simulink library "simpSubPlatform_cl"  (R2018b)
settings: Solver=VariableStepAuto  StartTime=0.0  StopTime=10.0  RelTol=1e-3
values from neighbouring files (symbols this model uses):
  CB2CMVec = [0 0 0]    [simpSubPlatform_ts.m]
  grav = 9.81    [simpSubPlatform_ts.m]
  inertiaMatrix = eye(3)    [simpSubPlatform_ts.m]
  initAngVel = [0 0 0]    [simpSubPlatform_ts.m]
  initEulerAngles = [0 0 0]    [simpSubPlatform_ts.m]
  initPos = [0 0 100]    [simpSubPlatform_ts.m]
  initVel = [0 0 0]    [simpSubPlatform_ts.m]
  m = mass    (= 2692.30769231)    [simpSubPlatform_ts.m]
  rho = 1000    [simpSubPlatform_ts.m]
  thr1Pt = [0 1 -.5]    [simpSubPlatform_ts.m]
  thr2Pt = [cosd(30),-sind(30),-.5]    [simpSubPlatform_ts.m]
  thr3Pt = [-cosd(30),-sind(30),-.5]    [simpSubPlatform_ts.m]
  vol = 3.5    [simpSubPlatform_ts.m]
undefined symbols (not defined in the file or in its folder): initAngRates, Jinv, sixDoFDynamics, sixDoFDynamics_ul
libraries: vrlib x5, eulAng2RotMat_ul x1
settings Model: Creator=Erin B  LastModifiedBy=Erin B

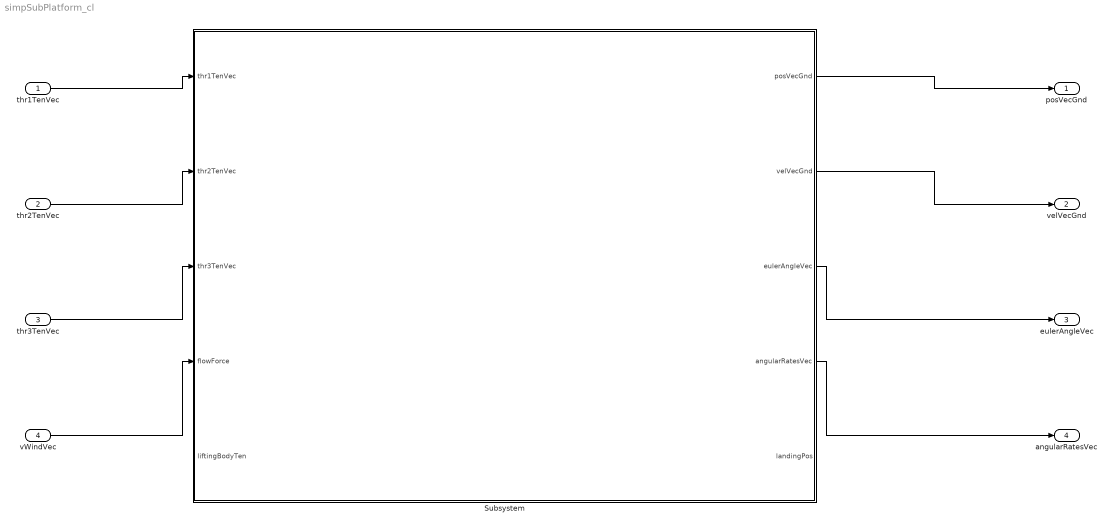
== system simpSubPlatform_cl ==
  thr1TenVec : Inport
  thr2TenVec : Inport  Port=2
  thr3TenVec : Inport  Port=3
  vWindVec : Inport  Port=4
  Subsystem : Subsystem
  posVecGnd : Outport
  velVecGnd : Outport  Port=2
  eulerAngleVec : Outport  Port=3
  angularRatesVec : Outport  Port=4
  wires:
  thr1TenVec/1 -> Subsystem/1(thr1TenVec)
  thr2TenVec/1 -> Subsystem/2(thr2TenVec)
  thr3TenVec/1 -> Subsystem/3(thr3TenVec)
  vWindVec/1 -> Subsystem/4(flowForce)
  Subsystem/1(posVecGnd) -> posVecGnd/1
  Subsystem/2(velVecGnd) -> velVecGnd/1
  Subsystem/3(eulerAngleVec) -> eulerAngleVec/1
  Subsystem/4(angularRatesVec) -> angularRatesVec/1

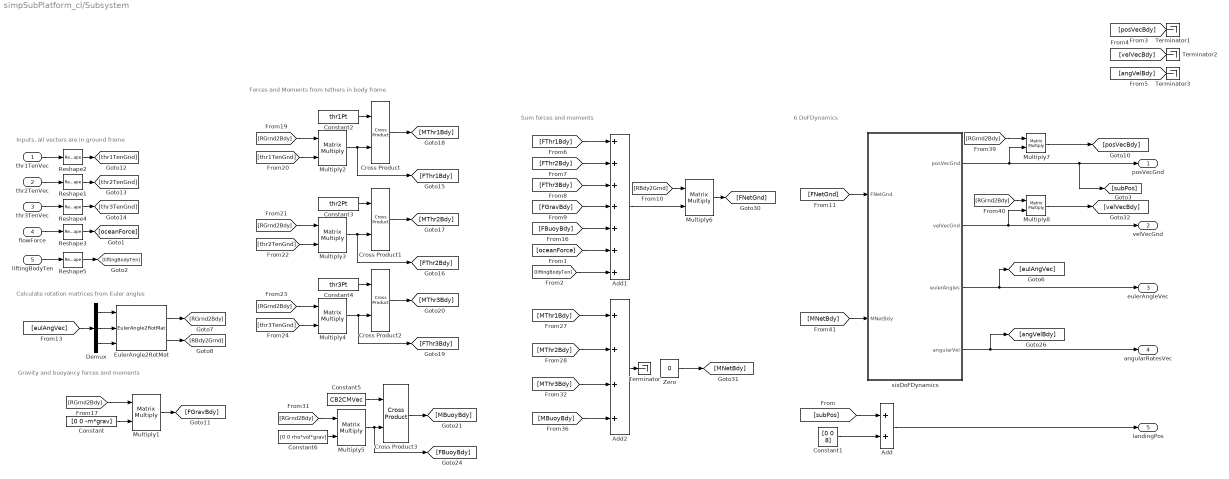
== system simpSubPlatform_cl/Subsystem ==
  note: Inputs, all vectors are in ground frame
  note: Calculate rotation matrices from Euler angles
  note: Gravity and buoyancy forces and moments
  note: Forces and Moments from tethers in body frame
  note: Sum forces and moments
  note: 6 DoFDynamics
  thr1TenVec : Inport
  thr2TenVec : Inport  Port=2
  thr3TenVec : Inport  Port=3
  flowForce : Inport  Port=4
  liftingBodyTen : Inport  Port=5
  Add : Sum
  Add1 : Sum  Inputs=+++++++
  Add2 : Sum  Inputs=++++
  Constant : Constant  Value=[0 0 -m*grav]
  Constant1 : Constant  Value=[0 0 8]
  Constant2 : Constant  Value=thr1Pt
  Constant3 : Constant  Value=thr2Pt
  Constant4 : Constant  Value=thr3Pt
  Constant5 : Constant  Value=CB2CMVec
  Constant6 : Constant  Value=[0 0 rho*vol*grav]
  Cross Product{,1..3} (4 alike) : vrlib/Utilities/Cross Product
      settings: SourceProductBaseCode=VR
  Demux : Demux  Outputs=3
  EulerAngle2RotMat : eulAng2RotMat_ul/EulerAngle2RotMat  SystemSampleTime=-1
  Multiply{1..8} (8 alike) : Product  Multiplication=Matrix(*)
  Reshape{1..5} (5 alike) : Reshape  OutputDimensionality=Column vector (2-D)
  Terminator{,1..3} (4 alike) : Terminator
  Zero : Constant  Value=0  OutDataTypeStr=Inherit: Inherit via back propagation
  sixDoFDynamics : Subsystem  AncestorBlock=sixDoFDynamics_ul/sixDoFDynamics  mask{m=m, initPos=initPos, initVel=initVel, J=inertiaMatrix, initEulAngs=initEulerAngles, initAngVel=initAngVel}
      mask prompts: m "Mass"; initPos "Initial position"; initVel "Initial velocity"; J "Inertia matrix"; initEulAngs "Initial Euler Angles"; initAngVel "Initial Angular Velocity Vec"
      mask init:
      | sixDoFDynamics_init
  posVecGnd : Outport
  velVecGnd : Outport  Port=2
  eulerAngleVec : Outport  Port=3
  angularRatesVec : Outport  Port=4
  landingPos : Outport  Port=5
  wires:
  [FThr1Bdy] -> Add1/1
  Multiply3/1 -> [FThr2Bdy], Cross Product1/2
  EulerAngle2RotMat/1 -> [RGrnd2Bdy]
  [MNetBdy] -> sixDoFDynamics/2(MNetBdy)
  [RGrnd2Bdy] -> Multiply8/1
  flowForce/1 -> Reshape3/1
  Reshape3/1 -> [oceanForce]
  [RGrnd2Bdy] -> Multiply7/1
  Constant5/1 -> Cross Product3/1
  thr1TenVec/1 -> Reshape2/1
  Reshape4/1 -> [thr3TenGnd]
  [eulAngVec] -> Demux/1
  [RGrnd2Bdy] -> Multiply3/1
  [RGrnd2Bdy] -> Multiply2/1
  Multiply5/1 -> Cross Product3/2, [FBuoyBdy]
  sixDoFDynamics/2(velVecGnd) -> velVecGnd/1, Multiply8/2
  [thr1TenGnd] -> Multiply2/2
  Multiply1/1 -> [FGravBdy]
  Add1/1 -> Multiply6/2
  sixDoFDynamics/3(eulerAngles) -> eulerAngleVec/1, [eulAngVec]
  Demux/2 -> EulerAngle2RotMat/2
  thr3TenVec/1 -> Reshape4/1
  [MThr2Bdy] -> Add2/2
  Multiply4/1 -> [FThr3Bdy], Cross Product2/2
  Demux/3 -> EulerAngle2RotMat/3
  sixDoFDynamics/1(posVecGnd) -> [subPos], posVecGnd/1, Multiply7/2
  sixDoFDynamics/4(angularVel) -> angularRatesVec/1, [angVelBdy]
  EulerAngle2RotMat/2 -> [RBdy2Grnd]
  Constant6/1 -> Multiply5/2
  [RGrnd2Bdy] -> Multiply5/1
  [MBuoyBdy] -> Add2/4
  [RBdy2Grnd] -> Multiply6/1
  Cross Product3/1 -> [MBuoyBdy]
  Reshape1/1 -> [thr2TenGnd]
  [FThr2Bdy] -> Add1/2
  Constant3/1 -> Cross Product1/1
  [FBuoyBdy] -> Add1/5
  Add2/1 -> Terminator/1
  Zero/1 -> [MNetBdy]
  Multiply2/1 -> [FThr1Bdy], Cross Product/2
  Constant2/1 -> Cross Product/1
  [MThr3Bdy] -> Add2/3
  Cross Product2/1 -> [MThr3Bdy]
  Cross Product/1 -> [MThr1Bdy]
  [thr2TenGnd] -> Multiply3/2
  Cross Product1/1 -> [MThr2Bdy]
  Constant/1 -> Multiply1/2
  [MThr1Bdy] -> Add2/1
  Multiply8/1 -> [velVecBdy]
  Reshape2/1 -> [thr1TenGnd]
  [FThr3Bdy] -> Add1/3
  [RGrnd2Bdy] -> Multiply4/1
  [thr3TenGnd] -> Multiply4/2
  Demux/1 -> EulerAngle2RotMat/1
  Constant4/1 -> Cross Product2/1
  [FNetGnd] -> sixDoFDynamics/1(FNetGnd)
  thr2TenVec/1 -> Reshape1/1
  Multiply7/1 -> [posVecBdy]
  [FGravBdy] -> Add1/4
  [RGrnd2Bdy] -> Multiply1/1
  [subPos] -> Add/1
  Constant1/1 -> Add/2
  Add/1 -> landingPos/1
  [oceanForce] -> Add1/6
  liftingBodyTen/1 -> Reshape5/1
  Reshape5/1 -> [liftingBodyTen]
  [liftingBodyTen] -> Add1/7
  Multiply6/1 -> [FNetGnd]

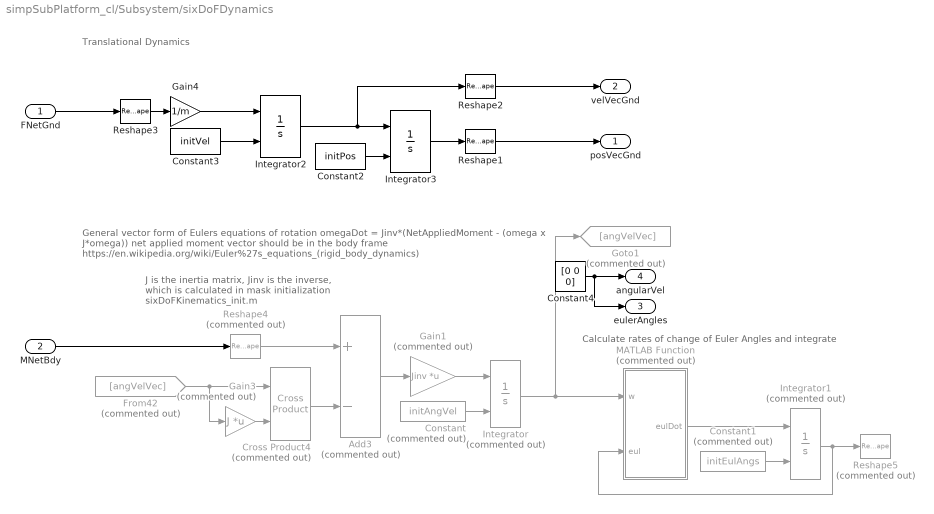
== system simpSubPlatform_cl/Subsystem/sixDoFDynamics ==
  note: J is the inertia matrix, Jinv is the inverse,
      | which is calculated in mask initialization
      | sixDoFKinematics_init.m
  note: General vector form of Eulers equations of rotation
      | omegaDot = Jinv*(NetAppliedMoment - (omega x J*omega))
      | net applied moment vector should be in the body frame
      | https://en.wikipedia.org/wiki/Euler%27s_equations_(rigid_body_dynamics)
  note: Calculate rates of change of Euler Angles and integrate
  note: Translational Dynamics
  FNetGnd : Inport
  MNetBdy : Inport  Port=2
  Add3 : Sum  Commented=on  Inputs=+-
  Constant : Constant  Commented=on  Value=initAngVel
  Constant1 : Constant  Commented=on  Value=initEulAngs
  Constant2 : Constant  Value=initPos
  Constant3 : Constant  Value=initVel
  Constant4 : Constant  Value=[0 0 0]
  Cross Product4 : vrlib/Utilities/Cross Product  Commented=on
      settings: SourceProductBaseCode=VR
  From42 : From  Commented=on  GotoTag=angVelVec
  Gain1 : Gain  Commented=on  Gain=Jinv  Multiplication=Matrix(K*u)
  Gain3 : Gain  Commented=on  Gain=J  Multiplication=Matrix(K*u)
  Gain4 : Gain  Gain=1/m
  Goto1 : Goto  Commented=on  GotoTag=angVelVec
  Integrator : Integrator  Commented=on  InitialConditionSource=external  InitialCondition=initAngRates
  Integrator1 : Integrator  Commented=on  InitialConditionSource=external  InitialCondition=initEulAngs
  Integrator2 : Integrator  InitialConditionSource=external  InitialCondition=initVel
  Integrator3 : Integrator  InitialConditionSource=external  InitialCondition=initPos
  MATLAB Function : MATLAB Function  Commented=on  TreatAsAtomicUnit=on
  Reshape1 : Reshape  OutputDimensionality=Column vector (2-D)
  Reshape2 : Reshape  OutputDimensionality=Column vector (2-D)
  Reshape3 : Reshape  OutputDimensionality=Column vector (2-D)
  Reshape4 : Reshape  Commented=on  OutputDimensionality=Column vector (2-D)
  Reshape5 : Reshape  Commented=on  OutputDimensionality=Column vector (2-D)
  posVecGnd : Outport
  velVecGnd : Outport  Port=2
  eulerAngles : Outport  Port=3
  angularVel : Outport  Port=4
  wires:
  Reshape4/1 -> Add3/1
  Reshape3/1 -> Gain4/1
  Reshape1/1 -> posVecGnd/1
  Reshape2/1 -> velVecGnd/1
  Constant3/1 -> Integrator2/2
  Constant2/1 -> Integrator3/2
  Constant1/1 -> Integrator1/2
  MATLAB Function/1(eulDot) -> Integrator1/1
  Constant/1 -> Integrator/2
  Integrator2/1 -> Integrator3/1, Reshape2/1
  Integrator3/1 -> Reshape1/1
  Gain4/1 -> Integrator2/1
  FNetGnd/1 -> Reshape3/1
  Cross Product4/1 -> Add3/2
  Gain1/1 -> Integrator/1
  Integrator1/1 -> MATLAB Function/2(eul), Reshape5/1
  Add3/1 -> Gain1/1
  Integrator/1 -> MATLAB Function/1(w), Goto1/1
  Gain3/1 -> Cross Product4/2
  From42/1 -> Gain3/1, Cross Product4/1
  MNetBdy/1 -> Reshape4/1
  Constant4/1 -> eulerAngles/1, angularVel/1

== matlab function simpSubPlatform_cl/Subsystem/sixDoFDynamics/MATLAB Function ==
  data: w input; eulDot output; eul input
function eulDot = fcn(w,eul)
% function that relates angular velocity vector to rates of change of Euler
% angles.
% w is angular velocity vector in body frame
% eul is vector of euler angles [roll, pitch, yaw]
eulDot = zeros(3,1);
eulDot(1) = w(1) + sin(eul(1))*tan(eul(2))*w(2) + cos(phi)*tan(eul(2))*w(3);
eulDot(2) = cos(ph)*w(2) - sin(ph)*w(3);...
eulDot(3) = sec(eul(2))*sin(ph)*w(2) + cos(ph)*sec(eul(2))*w(3);
end
